simulink model "c960x4096_x14_7_r2013b_frb"  (R2013b)
settings: Solver=ode45  StartTime=0.0  StopTime=40960  RelTol=1e-3
undefined symbols (not defined in the file): sfp
libraries: xbsIndex_r4 x14620, casper_library_misc x61, dspsigops x32, casper_library_multipliers x24, simulink x18, xps_library x18
(part 5 of 79)

== system c960x4096_x14_7_r2013b_frb/p0_scale ==
  sync : Inport
  S0 : Inport  Port=2
  S1 : Inport  Port=3
  S2 : Inport  Port=4
  S3 : Inport  Port=5
  S4 : Inport  Port=6
  S5 : Inport  Port=7
  S6 : Inport  Port=8
  S7 : Inport  Port=9
  SCALE : Inport  Port=10
  DocBlock : simulink/Model-Wide Utilities/DocBlock  DocumentType=Text
      content=|
      | - JMR, 04/30/13
      | Slice to separate the real and imaginary parts, apply the multiplicative
      | scale to each part, then cast down to Fix_8_5.
  Register{,1..3} (4 alike) : xbsIndex_r4/Register  init=0  rst=off  en=off  dbl_ovrd=off  block_type=register
  SCALE_Re_&_Im_0 : Subsystem
  SCALE_Re_&_Im_1 : Subsystem
  SCALE_Re_&_Im_2 : Subsystem
  SCALE_Re_&_Im_3 : Subsystem
  SCALE_Re_&_Im_4 : Subsystem
  SCALE_Re_&_Im_5 : Subsystem
  SCALE_Re_&_Im_6 : Subsystem
  SCALE_Re_&_Im_7 : Subsystem
  ri_to_c{1..8} (8 alike) : casper_library_misc/ri_to_c
  sync_out : Outport
  SO_out : Outport  Port=2
  S1_out : Outport  Port=3
  S2_out : Outport  Port=4
  S3_out : Outport  Port=5
  S4_out : Outport  Port=6
  S5_out : Outport  Port=7
  S6_out : Outport  Port=8
  S7_out : Outport  Port=9
  wires:
  ri_to_c7/1 -> S7_out/1
  ri_to_c6/1 -> S6_out/1
  ri_to_c5/1 -> S5_out/1
  ri_to_c4/1 -> S4_out/1
  ri_to_c3/1 -> S3_out/1
  ri_to_c2/1 -> S2_out/1
  ri_to_c1/1 -> S1_out/1
  ri_to_c8/1 -> SO_out/1
  Register/1 -> Register1/1
  SCALE/1 -> SCALE_Re_&_Im_7/2(SCALE), SCALE_Re_&_Im_6/2(SCALE), SCALE_Re_&_Im_5/2(SCALE), SCALE_Re_&_Im_4/2(SCALE), SCALE_Re_&_Im_3/2(SCALE), SCALE_Re_&_Im_2/2(SCALE), SCALE_Re_&_Im_1/2(SCALE), SCALE_Re_&_Im_0/2(SCALE)
  S7/1 -> SCALE_Re_&_Im_7/1(P_S)
  S6/1 -> SCALE_Re_&_Im_6/1(P_S)
  S5/1 -> SCALE_Re_&_Im_5/1(P_S)
  S4/1 -> SCALE_Re_&_Im_4/1(P_S)
  S3/1 -> SCALE_Re_&_Im_3/1(P_S)
  S2/1 -> SCALE_Re_&_Im_2/1(P_S)
  S1/1 -> SCALE_Re_&_Im_1/1(P_S)
  S0/1 -> SCALE_Re_&_Im_0/1(P_S)
  sync/1 -> Register/1
  SCALE_Re_&_Im_7/2(Im) -> ri_to_c7/2
  SCALE_Re_&_Im_7/1(Re) -> ri_to_c7/1
  SCALE_Re_&_Im_6/2(Im) -> ri_to_c6/2
  SCALE_Re_&_Im_6/1(Re) -> ri_to_c6/1
  SCALE_Re_&_Im_5/2(Im) -> ri_to_c5/2
  SCALE_Re_&_Im_5/1(Re) -> ri_to_c5/1
  SCALE_Re_&_Im_4/2(Im) -> ri_to_c4/2
  SCALE_Re_&_Im_4/1(Re) -> ri_to_c4/1
  SCALE_Re_&_Im_3/2(Im) -> ri_to_c3/2
  SCALE_Re_&_Im_3/1(Re) -> ri_to_c3/1
  SCALE_Re_&_Im_2/2(Im) -> ri_to_c2/2
  SCALE_Re_&_Im_2/1(Re) -> ri_to_c2/1
  SCALE_Re_&_Im_1/2(Im) -> ri_to_c1/2
  SCALE_Re_&_Im_1/1(Re) -> ri_to_c1/1
  SCALE_Re_&_Im_0/2(Im) -> ri_to_c8/2
  SCALE_Re_&_Im_0/1(Re) -> ri_to_c8/1
  Register1/1 -> Register2/1
  Register2/1 -> Register3/1
  Register3/1 -> sync_out/1

== system c960x4096_x14_7_r2013b_frb/p1_adc ==
  Band-Limited White Noise : simulink/Sources/Band-Limited White Noise  Cov=[0.1]  Ts=0.1  seed=[23341]
  Delay{1..16} (16 alike) : xbsIndex_r4/Delay  rst=off  infoeditControl=Selection of Reset will increase slice count due to use of real FFs and instead of SRLs  en=off  latency=2  dbl_ovrd=off  reg_retiming=on  block_type=delay
      settings: block_version=11.4
  Pulse Generator : DiscretePulseGenerator  Period=10  PulseWidth=5
  Register44 : xbsIndex_r4/Register  init=0  rst=off  en=off  dbl_ovrd=off  block_type=register
      settings: block_version=11.4
  Slice10 : xbsIndex_r4/Slice  nbits=1  boolean_output=on  mode=Lower Bit Location + Width  bit1=0  base1=MSB of Input  bit0=0  base0=LSB of Input  dbl_ovrd=off  block_type=slice
      settings: infoedit="Extracts a given range of bits from each input sample and presents it at the output.  The output type is ordinarily unsigned with binary point at zero, but can be Boolean when the slice is one bit wide.<P><P>Hardware notes: In hardware this block costs nothing."  block_version=10.1.3
  Subsystem1 : Subsystem
  asiaa_adc5g1 : Subsystem  Tag=xps:adc5g  AncestorBlock=xps_library/ADCs/asiaa_adc5g  mask(adc5g){input_mode=One-channel -- A, adc_brd=ZDOK 1, demux=1:1, adc_bit_width=8, adc_clk_rate=960, using_ctrl=on, test_ramp=off}
      mask prompts: input_mode "Input mode:"; adc_brd "ADC Board"; demux "Internal demux"; adc_bit_width "ADC Resolution (bits):"; adc_clk_rate "ADC Clock Rate (MHz):"; using_ctrl "use control"; test_ramp "start in test ramp mode"
      mask help:
      | Interface for the ASIAA 5 GSps ADC. Supports interleaving all four
      | cores using either input A or C, or interleaving two-cores each for
      | A and C. The hardware itself comes in two versions:
      |
      | DMUX 1:2 -- 4-bit samples, 4 parallel streams
      | DMUX 1:1 -- 8-bit samples, 2 parallel streams
      |
      | In either configuration this block will output 8 parallel streams
      | but the underlying interface, and the bitwidth of the samples,
      | will be different.
      mask init: same as c960x4096_x14_7_r2013b_frb/p0_adc/asiaa_adc5g1
      mask TypeOptions input_mode: One-channel -- A | One-channel -- C | Two-channel -- A&C
      mask TypeOptions adc_brd: ZDOK 0 | ZDOK 1
      mask TypeOptions demux: 1:1 | 1:2
      mask Callback demux:
      | demux = get_param(gcb,'demux');
      | if(strcmp(demux,'1:1')),
      |     set_param(gcb, 'adc_bit_width', '8')
      | elseif(strcmp(demux, '1:2')),
      |     set_param(gcb, 'adc_bit_width', '4');
      | else
      | end
  P0_DS : Outport
  1PPS : Outport  Port=2
  wires:
  Slice10/1 -> 1PPS/1
  asiaa_adc5g1/17(sync_out) -> Register44/1
  Register44/1 -> Slice10/1
  asiaa_adc5g1/1(a0) -> Delay5/1
  Delay5/1 -> Subsystem1/1(In1)
  asiaa_adc5g1/2(a1) -> Delay14/1
  Delay14/1 -> Subsystem1/2(In2)
  asiaa_adc5g1/3(a2) -> Delay1/1
  Delay1/1 -> Subsystem1/3(In3)
  asiaa_adc5g1/4(a3) -> Delay2/1
  Delay2/1 -> Subsystem1/4(In4)
  asiaa_adc5g1/5(a4) -> Delay3/1
  Delay3/1 -> Subsystem1/5(In5)
  asiaa_adc5g1/6(a5) -> Delay4/1
  Delay4/1 -> Subsystem1/6(In6)
  asiaa_adc5g1/7(a6) -> Delay6/1
  Delay6/1 -> Subsystem1/7(In7)
  asiaa_adc5g1/8(a7) -> Delay7/1
  Delay7/1 -> Subsystem1/8(In8)
  asiaa_adc5g1/9(a8) -> Delay8/1
  Delay8/1 -> Subsystem1/9(In9)
  asiaa_adc5g1/10(a9) -> Delay9/1
  Delay9/1 -> Subsystem1/10(In10)
  asiaa_adc5g1/11(a10) -> Delay10/1
  Delay10/1 -> Subsystem1/11(In11)
  asiaa_adc5g1/12(a11) -> Delay11/1
  Delay11/1 -> Subsystem1/12(In12)
  asiaa_adc5g1/13(a12) -> Delay12/1
  Delay12/1 -> Subsystem1/13(In13)
  asiaa_adc5g1/14(a13) -> Delay13/1
  Delay13/1 -> Subsystem1/14(In14)
  asiaa_adc5g1/15(a14) -> Delay15/1
  Delay15/1 -> Subsystem1/15(In15)
  asiaa_adc5g1/16(a15) -> Delay16/1
  Delay16/1 -> Subsystem1/16(In16)
  Subsystem1/1(Out1) -> P0_DS/1
  Band-Limited White Noise/1 -> asiaa_adc5g1/1(sim_a)
  Pulse Generator/1 -> asiaa_adc5g1/2(sim_sync)

== system c960x4096_x14_7_r2013b_frb/p1_scale ==
  sync : Inport
  S0 : Inport  Port=2
  S1 : Inport  Port=3
  S2 : Inport  Port=4
  S3 : Inport  Port=5
  S4 : Inport  Port=6
  S5 : Inport  Port=7
  S6 : Inport  Port=8
  S7 : Inport  Port=9
  SCALE : Inport  Port=10
  Delay3 : xbsIndex_r4/Delay  rst=off  infoeditControl=Selection of Reset will increase slice count due to use of real FFs and instead of SRLs  en=off  latency=4  dbl_ovrd=off  reg_retiming=off  block_type=delay
  DocBlock : simulink/Model-Wide Utilities/DocBlock  DocumentType=Text
      content=|
      | - JMR, 04/30/13
      | Placed original FFT green block inside this subsystem to reverse the 'sync'
      | and 'shift' inputs so that they connected directly in the next level above.
  SCALE_Re_&_Im_0 : Subsystem
  SCALE_Re_&_Im_1 : Subsystem
  SCALE_Re_&_Im_2 : Subsystem
  SCALE_Re_&_Im_3 : Subsystem
  SCALE_Re_&_Im_4 : Subsystem
  SCALE_Re_&_Im_5 : Subsystem
  SCALE_Re_&_Im_6 : Subsystem
  SCALE_Re_&_Im_7 : Subsystem
  ri_to_c{1..8} (8 alike) : casper_library_misc/ri_to_c
  sync_out : Outport
  SO_out : Outport  Port=2
  S1_out : Outport  Port=3
  S2_out : Outport  Port=4
  S3_out : Outport  Port=5
  S4_out : Outport  Port=6
  S5_out : Outport  Port=7
  S6_out : Outport  Port=8
  S7_out : Outport  Port=9
  wires:
  ri_to_c7/1 -> S7_out/1
  ri_to_c6/1 -> S6_out/1
  ri_to_c5/1 -> S5_out/1
  ri_to_c4/1 -> S4_out/1
  ri_to_c3/1 -> S3_out/1
  ri_to_c2/1 -> S2_out/1
  ri_to_c1/1 -> S1_out/1
  ri_to_c8/1 -> SO_out/1
  Delay3/1 -> sync_out/1
  SCALE/1 -> SCALE_Re_&_Im_7/2(SCALE), SCALE_Re_&_Im_6/2(SCALE), SCALE_Re_&_Im_5/2(SCALE), SCALE_Re_&_Im_4/2(SCALE), SCALE_Re_&_Im_3/2(SCALE), SCALE_Re_&_Im_2/2(SCALE), SCALE_Re_&_Im_1/2(SCALE), SCALE_Re_&_Im_0/2(SCALE)
  S7/1 -> SCALE_Re_&_Im_7/1(P_S)
  S6/1 -> SCALE_Re_&_Im_6/1(P_S)
  S5/1 -> SCALE_Re_&_Im_5/1(P_S)
  S4/1 -> SCALE_Re_&_Im_4/1(P_S)
  S3/1 -> SCALE_Re_&_Im_3/1(P_S)
  S2/1 -> SCALE_Re_&_Im_2/1(P_S)
  S1/1 -> SCALE_Re_&_Im_1/1(P_S)
  S0/1 -> SCALE_Re_&_Im_0/1(P_S)
  sync/1 -> Delay3/1
  SCALE_Re_&_Im_7/2(Im) -> ri_to_c7/2
  SCALE_Re_&_Im_7/1(Re) -> ri_to_c7/1
  SCALE_Re_&_Im_6/2(Im) -> ri_to_c6/2
  SCALE_Re_&_Im_6/1(Re) -> ri_to_c6/1
  SCALE_Re_&_Im_5/2(Im) -> ri_to_c5/2
  SCALE_Re_&_Im_5/1(Re) -> ri_to_c5/1
  SCALE_Re_&_Im_4/2(Im) -> ri_to_c4/2
  SCALE_Re_&_Im_4/1(Re) -> ri_to_c4/1
  SCALE_Re_&_Im_3/2(Im) -> ri_to_c3/2
  SCALE_Re_&_Im_3/1(Re) -> ri_to_c3/1
  SCALE_Re_&_Im_2/2(Im) -> ri_to_c2/2
  SCALE_Re_&_Im_2/1(Re) -> ri_to_c2/1
  SCALE_Re_&_Im_1/2(Im) -> ri_to_c1/2
  SCALE_Re_&_Im_1/1(Re) -> ri_to_c1/1
  SCALE_Re_&_Im_0/2(Im) -> ri_to_c8/2
  SCALE_Re_&_Im_0/1(Re) -> ri_to_c8/1

== system c960x4096_x14_7_r2013b_frb/plat_bd ==
  out_reg : Inport
  assert_reg : xbsIndex_r4/Assert  assert_type=on  type_source=Explicitly  gui_display_data_type=Fixed-point  arith_type=Unsigned  n_bits=32  bin_pt=0  preci_type=Single  exp_width=8  frac_width=24  assert_rate=off  rate_source=Explicitly  period=1  output_port=on  block_type=assert
  c960x4096_x14_7_frbout_plat_bd_user_data_in : xbsIndex_r4/Gateway Out  inherit_from_input=off  hdl_port=on  timing_constraint=None  locs_specified=off  LOCs={}  UseAsDAC=off  DACChannel='1'  block_type=gatewayout
  cast_gw : xbsIndex_r4/Convert  gui_display_data_type=Fixed-point  arith_type=Unsigned  n_bits=32  bin_pt=0  float_type=Single  exp_bits=8  fraction_bits=24  quantization=Truncate  overflow=Wrap  en=off  latency=0  dbl_ovrd=off  pipeline=off  block_type=convert
  io_delay : xbsIndex_r4/Delay  rst=off  infoeditControl=Selection of Reset will increase slice count due to use of real FFs and instead of SRLs  en=off  latency=0  dbl_ovrd=off  reg_retiming=on  block_type=delay
  reint1 : xbsIndex_r4/Reinterpret  force_arith_type=on  arith_type=Unsigned  force_bin_pt=on  bin_pt=0  block_type=reinterpret
  sim_out : Outport
  wires:
  io_delay/1 -> cast_gw/1
  cast_gw/1 -> c960x4096_x14_7_frbout_plat_bd_user_data_in/1
  c960x4096_x14_7_frbout_plat_bd_user_data_in/1 -> sim_out/1
  out_reg/1 -> assert_reg/1
  assert_reg/1 -> reint1/1
  reint1/1 -> io_delay/1

== system c960x4096_x14_7_r2013b_frb/pt_0 ==
  sim_1 : Inport
  c960x4096_x14_7_frbout_pt_0_user_data_out : xbsIndex_r4/Gateway In  gui_display_data_type=Fixed-point  arith_type=Unsigned  n_bits=32  bin_pt=0  preci_type=Single  exp_width=8  frac_width=24  quantization="Round  (unbiased: +/- Inf)"  overflow=Saturate  period=1  dbl_ovrd=off  timing_constraint=None  locs_specified=off  LOCs={}  UseAsADC=off  ADCChannel='1'  inherit_from_input=off  hdl_port=on  block_type=gatewayin
  io_delay : xbsIndex_r4/Delay  rst=off  infoeditControl=Selection of Reset will increase slice count due to use of real FFs and instead of SRLs  en=off  latency=0  dbl_ovrd=off  reg_retiming=on  block_type=delay
  reint1 : xbsIndex_r4/Reinterpret  force_arith_type=on  arith_type=Unsigned  force_bin_pt=on  bin_pt=0  block_type=reinterpret
  slice_reg : xbsIndex_r4/Slice  nbits=16  boolean_output=off  mode=Lower Bit Location + Width  bit1=0  base1=MSB of Input  bit0=0  base0=LSB of Input  dbl_ovrd=off  block_type=slice
  in_reg : Outport
  wires:
  c960x4096_x14_7_frbout_pt_0_user_data_out/1 -> io_delay/1
  sim_1/1 -> c960x4096_x14_7_frbout_pt_0_user_data_out/1
  io_delay/1 -> slice_reg/1
  slice_reg/1 -> reint1/1
  reint1/1 -> in_reg/1

== system c960x4096_x14_7_r2013b_frb/pt_1 ==
  sim_1 : Inport
  c960x4096_x14_7_frbout_pt_1_user_data_out : xbsIndex_r4/Gateway In  gui_display_data_type=Fixed-point  arith_type=Unsigned  n_bits=32  bin_pt=0  preci_type=Single  exp_width=8  frac_width=24  quantization="Round  (unbiased: +/- Inf)"  overflow=Saturate  period=1  dbl_ovrd=off  timing_constraint=None  locs_specified=off  LOCs={}  UseAsADC=off  ADCChannel='1'  inherit_from_input=off  hdl_port=on  block_type=gatewayin
  io_delay : xbsIndex_r4/Delay  rst=off  infoeditControl=Selection of Reset will increase slice count due to use of real FFs and instead of SRLs  en=off  latency=0  dbl_ovrd=off  reg_retiming=on  block_type=delay
  reint1 : xbsIndex_r4/Reinterpret  force_arith_type=on  arith_type=Unsigned  force_bin_pt=on  bin_pt=0  block_type=reinterpret
  slice_reg : xbsIndex_r4/Slice  nbits=16  boolean_output=off  mode=Lower Bit Location + Width  bit1=0  base1=MSB of Input  bit0=0  base0=LSB of Input  dbl_ovrd=off  block_type=slice
  in_reg : Outport
  wires:
  c960x4096_x14_7_frbout_pt_1_user_data_out/1 -> io_delay/1
  sim_1/1 -> c960x4096_x14_7_frbout_pt_1_user_data_out/1
  io_delay/1 -> slice_reg/1
  slice_reg/1 -> reint1/1
  reint1/1 -> in_reg/1

== system c960x4096_x14_7_r2013b_frb/pt_2 ==
  sim_1 : Inport
  c960x4096_x14_7_frbout_pt_2_user_data_out : xbsIndex_r4/Gateway In  gui_display_data_type=Fixed-point  arith_type=Unsigned  n_bits=32  bin_pt=0  preci_type=Single  exp_width=8  frac_width=24  quantization="Round  (unbiased: +/- Inf)"  overflow=Saturate  period=1  dbl_ovrd=off  timing_constraint=None  locs_specified=off  LOCs={}  UseAsADC=off  ADCChannel='1'  inherit_from_input=off  hdl_port=on  block_type=gatewayin
  io_delay : xbsIndex_r4/Delay  rst=off  infoeditControl=Selection of Reset will increase slice count due to use of real FFs and instead of SRLs  en=off  latency=0  dbl_ovrd=off  reg_retiming=on  block_type=delay
  reint1 : xbsIndex_r4/Reinterpret  force_arith_type=on  arith_type=Unsigned  force_bin_pt=on  bin_pt=0  block_type=reinterpret
  slice_reg : xbsIndex_r4/Slice  nbits=16  boolean_output=off  mode=Lower Bit Location + Width  bit1=0  base1=MSB of Input  bit0=0  base0=LSB of Input  dbl_ovrd=off  block_type=slice
  in_reg : Outport
  wires:
  c960x4096_x14_7_frbout_pt_2_user_data_out/1 -> io_delay/1
  sim_1/1 -> c960x4096_x14_7_frbout_pt_2_user_data_out/1
  io_delay/1 -> slice_reg/1
  slice_reg/1 -> reint1/1
  reint1/1 -> in_reg/1

== system c960x4096_x14_7_r2013b_frb/pt_3 ==
  sim_1 : Inport
  c960x4096_x14_7_frbout_pt_3_user_data_out : xbsIndex_r4/Gateway In  gui_display_data_type=Fixed-point  arith_type=Unsigned  n_bits=32  bin_pt=0  preci_type=Single  exp_width=8  frac_width=24  quantization="Round  (unbiased: +/- Inf)"  overflow=Saturate  period=1  dbl_ovrd=off  timing_constraint=None  locs_specified=off  LOCs={}  UseAsADC=off  ADCChannel='1'  inherit_from_input=off  hdl_port=on  block_type=gatewayin
  io_delay : xbsIndex_r4/Delay  rst=off  infoeditControl=Selection of Reset will increase slice count due to use of real FFs and instead of SRLs  en=off  latency=0  dbl_ovrd=off  reg_retiming=on  block_type=delay
  reint1 : xbsIndex_r4/Reinterpret  force_arith_type=on  arith_type=Unsigned  force_bin_pt=on  bin_pt=0  block_type=reinterpret
  slice_reg : xbsIndex_r4/Slice  nbits=16  boolean_output=off  mode=Lower Bit Location + Width  bit1=0  base1=MSB of Input  bit0=0  base0=LSB of Input  dbl_ovrd=off  block_type=slice
  in_reg : Outport
  wires:
  c960x4096_x14_7_frbout_pt_3_user_data_out/1 -> io_delay/1
  sim_1/1 -> c960x4096_x14_7_frbout_pt_3_user_data_out/1
  io_delay/1 -> slice_reg/1
  slice_reg/1 -> reint1/1
  reint1/1 -> in_reg/1

== system c960x4096_x14_7_r2013b_frb/pt_4 ==
  sim_1 : Inport
  c960x4096_x14_7_frbout_pt_4_user_data_out : xbsIndex_r4/Gateway In  gui_display_data_type=Fixed-point  arith_type=Unsigned  n_bits=32  bin_pt=0  preci_type=Single  exp_width=8  frac_width=24  quantization="Round  (unbiased: +/- Inf)"  overflow=Saturate  period=1  dbl_ovrd=off  timing_constraint=None  locs_specified=off  LOCs={}  UseAsADC=off  ADCChannel='1'  inherit_from_input=off  hdl_port=on  block_type=gatewayin
  io_delay : xbsIndex_r4/Delay  rst=off  infoeditControl=Selection of Reset will increase slice count due to use of real FFs and instead of SRLs  en=off  latency=0  dbl_ovrd=off  reg_retiming=on  block_type=delay
  reint1 : xbsIndex_r4/Reinterpret  force_arith_type=on  arith_type=Unsigned  force_bin_pt=on  bin_pt=0  block_type=reinterpret
  slice_reg : xbsIndex_r4/Slice  nbits=16  boolean_output=off  mode=Lower Bit Location + Width  bit1=0  base1=MSB of Input  bit0=0  base0=LSB of Input  dbl_ovrd=off  block_type=slice
  in_reg : Outport
  wires:
  c960x4096_x14_7_frbout_pt_4_user_data_out/1 -> io_delay/1
  sim_1/1 -> c960x4096_x14_7_frbout_pt_4_user_data_out/1
  io_delay/1 -> slice_reg/1
  slice_reg/1 -> reint1/1
  reint1/1 -> in_reg/1

== system c960x4096_x14_7_r2013b_frb/pt_5 ==
  sim_1 : Inport
  c960x4096_x14_7_frbout_pt_5_user_data_out : xbsIndex_r4/Gateway In  gui_display_data_type=Fixed-point  arith_type=Unsigned  n_bits=32  bin_pt=0  preci_type=Single  exp_width=8  frac_width=24  quantization="Round  (unbiased: +/- Inf)"  overflow=Saturate  period=1  dbl_ovrd=off  timing_constraint=None  locs_specified=off  LOCs={}  UseAsADC=off  ADCChannel='1'  inherit_from_input=off  hdl_port=on  block_type=gatewayin
  io_delay : xbsIndex_r4/Delay  rst=off  infoeditControl=Selection of Reset will increase slice count due to use of real FFs and instead of SRLs  en=off  latency=0  dbl_ovrd=off  reg_retiming=on  block_type=delay
  reint1 : xbsIndex_r4/Reinterpret  force_arith_type=on  arith_type=Unsigned  force_bin_pt=on  bin_pt=0  block_type=reinterpret
  slice_reg : xbsIndex_r4/Slice  nbits=16  boolean_output=off  mode=Lower Bit Location + Width  bit1=0  base1=MSB of Input  bit0=0  base0=LSB of Input  dbl_ovrd=off  block_type=slice
  in_reg : Outport
  wires:
  c960x4096_x14_7_frbout_pt_5_user_data_out/1 -> io_delay/1
  sim_1/1 -> c960x4096_x14_7_frbout_pt_5_user_data_out/1
  io_delay/1 -> slice_reg/1
  slice_reg/1 -> reint1/1
  reint1/1 -> in_reg/1

== system c960x4096_x14_7_r2013b_frb/pt_6 ==
  sim_1 : Inport
  c960x4096_x14_7_frbout_pt_6_user_data_out : xbsIndex_r4/Gateway In  gui_display_data_type=Fixed-point  arith_type=Unsigned  n_bits=32  bin_pt=0  preci_type=Single  exp_width=8  frac_width=24  quantization="Round  (unbiased: +/- Inf)"  overflow=Saturate  period=1  dbl_ovrd=off  timing_constraint=None  locs_specified=off  LOCs={}  UseAsADC=off  ADCChannel='1'  inherit_from_input=off  hdl_port=on  block_type=gatewayin
  io_delay : xbsIndex_r4/Delay  rst=off  infoeditControl=Selection of Reset will increase slice count due to use of real FFs and instead of SRLs  en=off  latency=0  dbl_ovrd=off  reg_retiming=on  block_type=delay
  reint1 : xbsIndex_r4/Reinterpret  force_arith_type=on  arith_type=Unsigned  force_bin_pt=on  bin_pt=0  block_type=reinterpret
  slice_reg : xbsIndex_r4/Slice  nbits=16  boolean_output=off  mode=Lower Bit Location + Width  bit1=0  base1=MSB of Input  bit0=0  base0=LSB of Input  dbl_ovrd=off  block_type=slice
  in_reg : Outport
  wires:
  c960x4096_x14_7_frbout_pt_6_user_data_out/1 -> io_delay/1
  sim_1/1 -> c960x4096_x14_7_frbout_pt_6_user_data_out/1
  io_delay/1 -> slice_reg/1
  slice_reg/1 -> reint1/1
  reint1/1 -> in_reg/1

== system c960x4096_x14_7_r2013b_frb/pt_7 ==
  sim_1 : Inport
  c960x4096_x14_7_frbout_pt_7_user_data_out : xbsIndex_r4/Gateway In  gui_display_data_type=Fixed-point  arith_type=Unsigned  n_bits=32  bin_pt=0  preci_type=Single  exp_width=8  frac_width=24  quantization="Round  (unbiased: +/- Inf)"  overflow=Saturate  period=1  dbl_ovrd=off  timing_constraint=None  locs_specified=off  LOCs={}  UseAsADC=off  ADCChannel='1'  inherit_from_input=off  hdl_port=on  block_type=gatewayin
  io_delay : xbsIndex_r4/Delay  rst=off  infoeditControl=Selection of Reset will increase slice count due to use of real FFs and instead of SRLs  en=off  latency=0  dbl_ovrd=off  reg_retiming=on  block_type=delay
  reint1 : xbsIndex_r4/Reinterpret  force_arith_type=on  arith_type=Unsigned  force_bin_pt=on  bin_pt=0  block_type=reinterpret
  slice_reg : xbsIndex_r4/Slice  nbits=16  boolean_output=off  mode=Lower Bit Location + Width  bit1=0  base1=MSB of Input  bit0=0  base0=LSB of Input  dbl_ovrd=off  block_type=slice
  in_reg : Outport
  wires:
  c960x4096_x14_7_frbout_pt_7_user_data_out/1 -> io_delay/1
  sim_1/1 -> c960x4096_x14_7_frbout_pt_7_user_data_out/1
  io_delay/1 -> slice_reg/1
  slice_reg/1 -> reint1/1
  reint1/1 -> in_reg/1

== system c960x4096_x14_7_r2013b_frb/reset ==
  sim_1 : Inport
  c960x4096_x14_7_frbout_reset_user_data_out : xbsIndex_r4/Gateway In  gui_display_data_type=Fixed-point  arith_type=Unsigned  n_bits=32  bin_pt=0  preci_type=Single  exp_width=8  frac_width=24  quantization="Round  (unbiased: +/- Inf)"  overflow=Saturate  period=1  dbl_ovrd=off  timing_constraint=None  locs_specified=off  LOCs={}  UseAsADC=off  ADCChannel='1'  inherit_from_input=off  hdl_port=on  block_type=gatewayin
  io_delay : xbsIndex_r4/Delay  rst=off  infoeditControl=Selection of Reset will increase slice count due to use of real FFs and instead of SRLs  en=off  latency=0  dbl_ovrd=off  reg_retiming=on  block_type=delay
  reint1 : xbsIndex_r4/Reinterpret  force_arith_type=on  arith_type=Unsigned  force_bin_pt=on  bin_pt=0  block_type=reinterpret
  slice_reg : xbsIndex_r4/Slice  nbits=32  boolean_output=off  mode=Lower Bit Location + Width  bit1=0  base1=MSB of Input  bit0=0  base0=LSB of Input  dbl_ovrd=off  block_type=slice
  in_reg : Outport
  wires:
  c960x4096_x14_7_frbout_reset_user_data_out/1 -> io_delay/1
  sim_1/1 -> c960x4096_x14_7_frbout_reset_user_data_out/1
  io_delay/1 -> slice_reg/1
  slice_reg/1 -> reint1/1
  reint1/1 -> in_reg/1

== system c960x4096_x14_7_r2013b_frb/rst_cpoge ==
  sim_1 : Inport
  c960x4096_x14_7_frbout_rst_cpoge_user_data_out : xbsIndex_r4/Gateway In  gui_display_data_type=Fixed-point  arith_type=Unsigned  n_bits=32  bin_pt=0  preci_type=Single  exp_width=8  frac_width=24  quantization="Round  (unbiased: +/- Inf)"  overflow=Saturate  period=1  dbl_ovrd=off  timing_constraint=None  locs_specified=off  LOCs={}  UseAsADC=off  ADCChannel='1'  inherit_from_input=off  hdl_port=on  block_type=gatewayin
  io_delay : xbsIndex_r4/Delay  rst=off  infoeditControl=Selection of Reset will increase slice count due to use of real FFs and instead of SRLs  en=off  latency=0  dbl_ovrd=off  reg_retiming=on  block_type=delay
  reint1 : xbsIndex_r4/Reinterpret  force_arith_type=on  arith_type=Unsigned  force_bin_pt=on  bin_pt=0  block_type=reinterpret
  slice_reg : xbsIndex_r4/Slice  nbits=32  boolean_output=off  mode=Lower Bit Location + Width  bit1=0  base1=MSB of Input  bit0=0  base0=LSB of Input  dbl_ovrd=off  block_type=slice
  in_reg : Outport
  wires:
  c960x4096_x14_7_frbout_rst_cpoge_user_data_out/1 -> io_delay/1
  sim_1/1 -> c960x4096_x14_7_frbout_rst_cpoge_user_data_out/1
  io_delay/1 -> slice_reg/1
  slice_reg/1 -> reint1/1
  reint1/1 -> in_reg/1

== system c960x4096_x14_7_r2013b_frb/scale_p0 ==
  sim_1 : Inport
  c960x4096_x14_7_frbout_scale_p0_user_data_out : xbsIndex_r4/Gateway In  gui_display_data_type=Fixed-point  arith_type=Unsigned  n_bits=32  bin_pt=0  preci_type=Single  exp_width=8  frac_width=24  quantization="Round  (unbiased: +/- Inf)"  overflow=Saturate  period=1  dbl_ovrd=off  timing_constraint=None  locs_specified=off  LOCs={}  UseAsADC=off  ADCChannel='1'  inherit_from_input=off  hdl_port=on  block_type=gatewayin
  io_delay : xbsIndex_r4/Delay  rst=off  infoeditControl=Selection of Reset will increase slice count due to use of real FFs and instead of SRLs  en=off  latency=0  dbl_ovrd=off  reg_retiming=on  block_type=delay
  reint1 : xbsIndex_r4/Reinterpret  force_arith_type=on  arith_type=Unsigned  force_bin_pt=on  bin_pt=16  block_type=reinterpret
  slice_reg : xbsIndex_r4/Slice  nbits=32  boolean_output=off  mode=Lower Bit Location + Width  bit1=0  base1=MSB of Input  bit0=0  base0=LSB of Input  dbl_ovrd=off  block_type=slice
  in_reg : Outport
  wires:
  c960x4096_x14_7_frbout_scale_p0_user_data_out/1 -> io_delay/1
  sim_1/1 -> c960x4096_x14_7_frbout_scale_p0_user_data_out/1
  io_delay/1 -> slice_reg/1
  slice_reg/1 -> reint1/1
  reint1/1 -> in_reg/1

== system c960x4096_x14_7_r2013b_frb/scale_p1 ==
  sim_1 : Inport
  c960x4096_x14_7_frbout_scale_p1_user_data_out : xbsIndex_r4/Gateway In  gui_display_data_type=Fixed-point  arith_type=Unsigned  n_bits=32  bin_pt=0  preci_type=Single  exp_width=8  frac_width=24  quantization="Round  (unbiased: +/- Inf)"  overflow=Saturate  period=1  dbl_ovrd=off  timing_constraint=None  locs_specified=off  LOCs={}  UseAsADC=off  ADCChannel='1'  inherit_from_input=off  hdl_port=on  block_type=gatewayin
  io_delay : xbsIndex_r4/Delay  rst=off  infoeditControl=Selection of Reset will increase slice count due to use of real FFs and instead of SRLs  en=off  latency=0  dbl_ovrd=off  reg_retiming=on  block_type=delay
  reint1 : xbsIndex_r4/Reinterpret  force_arith_type=on  arith_type=Unsigned  force_bin_pt=on  bin_pt=16  block_type=reinterpret
  slice_reg : xbsIndex_r4/Slice  nbits=32  boolean_output=off  mode=Lower Bit Location + Width  bit1=0  base1=MSB of Input  bit0=0  base0=LSB of Input  dbl_ovrd=off  block_type=slice
  in_reg : Outport
  wires:
  c960x4096_x14_7_frbout_scale_p1_user_data_out/1 -> io_delay/1
  sim_1/1 -> c960x4096_x14_7_frbout_scale_p1_user_data_out/1
  io_delay/1 -> slice_reg/1
  slice_reg/1 -> reint1/1
  reint1/1 -> in_reg/1

== system c960x4096_x14_7_r2013b_frb/spec_tick_gen ==
  In : Inport
  Counter3 : xbsIndex_r4/Counter  cnt_type=Free Running  cnt_to=Inf  operation=Up  start_count=0  cnt_by_val=1  arith_type=Unsigned  n_bits=2  bin_pt=0  load_pin=off  rst=on  en=off  explicit_period=on  period=1  dbl_ovrd=off  use_behavioral_HDL=off  implementation=DSP48  block_type=counter
      settings: block_version=11.3
  Slice1 : xbsIndex_r4/Slice  nbits=1  boolean_output=on  mode=Lower Bit Location + Width  bit1=7  base1=MSB of Input  bit0=1  base0=LSB of Input  dbl_ovrd=off  block_type=slice
      settings: block_version=10.1.3
  edge_detect3 : Subsystem  AncestorBlock=casper_library_misc/edge_detect  mask(edge_detect){edge=Falling, polarity=Active High, x_in=[0 0.08 0.08 0.16 0.16 0.24 0.24 0.32 0.32 0.4], y_in=[1  1 -1 -1 -1 -1 -1 -1 -1 -1], x_out=[0.6 0.68 0.68 0.76 0.76 0.84 0.84 0.92 0.92 1], y_out=[-1 -1  1  1 -1 -1 -1 -1 -1 -1]}
      mask prompts: edge "Edge Type"; polarity "Output Polarity"; x_in "Input X Positions"; y_in "Input Y Positions"; x_out "Output X Positions"; y_out "Output Y Positions"
      mask help: Output is active for one-cycle after each edge of the specified type (i.e. rising, falling or both).
      mask init: same as c960x4096_x14_7_r2013b_frb/edge_detect2
      settings: AttributesFormatString=|
      | falling edges
      | active high
      mask Help: Output is active for one-cycle after each edge of the specified type (i.e. rising, falling, or both).  Latency is zero.
      mask TypeOptions edge: Rising | Falling | Both
      mask TypeOptions polarity: Active High | Active Low
      mask Display:
      | plot(x_in_num,0.5+y_in_num*0.2);
      | plot(x_out_num,0.5+y_out_num*0.2);
  Out : Outport
  wires:
  In/1 -> Counter3/1
  Counter3/1 -> Slice1/1
  Slice1/1 -> edge_detect3/1(in)
  edge_detect3/1(out) -> Out/1
